simulink model "controlSystem_PowerScope"  (R2021a)
settings: Solver=VariableStepAuto  StartTime=0.0  StopTime=50  RelTol=1e-7
undefined symbols (not defined in the file): initialFuel, maxEngineTemp, maxEngineTorque, maxMotorTemp, maxMotorTorque, maxRegenTorque, motorVoltage, sigbuilder_block
libraries: autolibshared x6, autolibsharedcoupling x3, autolibhevctrlrcommon x2, autolibutils x2, autolibmappedmotor x2, autolibshareddiff x1, autolibtransamt x1, autolibdcdc x1, autolibdatasheetbattery x1, autolibsharedmappedengines x1
(part 3 of 5)

== system controlSystem_PowerScope/Signal Builder ==
  Demux : Demux  Tag=STV Demux  Outputs=3
      settings: DisplayOption=none
  FromWs : FromWorkspace  Tag=STV FromWs  VariableName=tuvar
      SigBuilderData=|
      | common.afterFinalStr = 'Extrapolate'
      | common.sampleTime = 0
      | dataSet.timeRange = [0 50]
      | dataSet.name = 'Group 1'
      | sbobj.Groups.Name = 'Group 1'
      | sbobj.Groups.Signals(1).Name = 'Signal 1'
      | sbobj.Groups.Signals(1).XData = [0 5 5 50]
      | sbobj.Groups.Signals(1).YData = [0 0 1 1]
      | sbobj.Groups.Signals(2).Name = 'Signal 2'
      | sbobj.Groups.Signals(2).XData = [0 50]
      | sbobj.Groups.Signals(2).YData = [0 0]
      | sbobj.Groups.Signals(3).Name = 'Signal 3'
      | sbobj.Groups.Signals(3).XData = [0 5 10 20 25 50]
      | sbobj.Groups.Signals(3).YData = [0 0 1 1 0 0]
      | sbobj.Groups.TimeRange = [0 50]
  Signal 1 : Outport  Tag=STV Outport
  Signal 2 : Outport  Tag=STV Outport  Port=2
  Signal 3 : Outport  Tag=STV Outport  Port=3
  wires:
  Demux/1 -> Signal 1/1
  FromWs/1 -> Demux/1
  Demux/2 -> Signal 2/1
  Demux/3 -> Signal 3/1

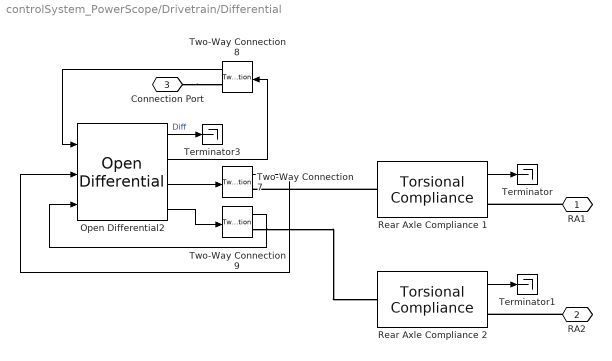
== system controlSystem_PowerScope/Drivetrain/Differential ==
  Open Differential2 : autolibshareddiff/Open Differential  DiffEffModelPopup=Constant  InterpMethod=Linear point-slope  extTamb=off  shaftSwitchMask=To the left of center-line  Ndiff=1  Jd=.025  bd=1e-3  Jw1=.01  bw1=1e-3  Jw2=.01  bw2=1e-3  omegaw1o=0  omegaw2o=0  eta=1  eta_tbl=reshape([0.64 0.76 0.8 0.81 0.83 0.84 0.84 0.56 0.73 0.78 0.8 0.83 0.84 0.84 0.54 0.71 0.77 0.8 0.82 0.84 0.84 0.53 0.71 0.77 0.8 0.83 0.84 0.84 0.51 0.71 0.77 0.8 0.83 0.84 0.85 0.52 0.7 0.77 0.8 0.83 0.84 0.85 0.51 0.71 0.76 0.79 0.83 0.84 0.85 0.5 0.69 0.76 0.79 0.82 0.84 0.85 0.45 0.68 0.75 0.78 0.82 0.84 0.85 0.43 0.67 0.74 0.78 0.81 0.83 0.84 0.38 0.63 0.71 0.75 0.8 0.82 0.83 0.81 0.86 0.88 0.89 0.89 0.89 0.9 0.77 0.85 0.87 0.88 0.89 0.9 0.9 0.72 0.82 0.86 0.87 0.88 0.89 0.9 0.68 0.8 0.84 0.86 0.88 0.89 0.89 0.67 0.8 0.84 0.86 0.88 0.89 0.9 0.67 0.8 0.84 0.86 0.88 0.89 0.9 0.65 0.8 0.84 0.86 0.88 0.89 0.9 0.64 0.79 0.83 0.86 0.88 0.89 0.9 0.63 0.78 0.83 0.86 0.88 0.89 0.9 0.59 0.76 0.82 0.85 0.87 0.89 0.9 0.53 0.73 0.8 0.83 0.86 0.88 0.89], 7, 11, 2)  Trq_bpts=[25, 50, 75, 100, 150, 200, 250]  omega_bpts=[52.4 78.5 105 131 157 183 209 262 314 419 524]  Temp_bpts=[290 358]  Tamb=297.15  maxAbsSpd=5e3  aMode=1
      settings: SourceProductBaseCode=PW,DR,MT,UV,VE
  Rear Axle Compliance 1 : autolibsharedcoupling/Torsional Compliance  port_config=Two-way connection  extInfo=on  k=1e4  b=1e2  theta_o=0  domega_o=0  omega_c=3000  blkID=0  aMode=1
      settings: SourceProductBaseCode=PW,DR,MT,UV,VE
  Rear Axle Compliance 2 : autolibsharedcoupling/Torsional Compliance  port_config=Two-way connection  extInfo=on  k=1e4  b=1e2  theta_o=0  domega_o=0  omega_c=3000  blkID=0  aMode=1
      settings: SourceProductBaseCode=PW,DR,MT,UV,VE
  Terminator : Terminator
  Terminator1 : Terminator
  Terminator3 : Terminator
  Two-Way Connection7 : TwoWayConnection
  Two-Way Connection8 : TwoWayConnection
  Two-Way Connection9 : TwoWayConnection
  RA1 : PMIOPort  Side=Right
  RA2 : PMIOPort  Port=2  Side=Right
  Connection Port : PMIOPort  Port=3  Side=Left
  wires:
  Open Differential2/4 -> Two-Way Connection9/1
  Open Differential2/1 -> Terminator3/1  "Diff"
  Open Differential2/2 -> Two-Way Connection8/1
  Two-Way Connection7/1 -> Open Differential2/2
  Two-Way Connection9/1 -> Open Differential2/3
  Two-Way Connection8/1 -> Open Differential2/1
  Open Differential2/3 -> Two-Way Connection7/1
  Rear Axle Compliance 1/1 -> Terminator/1
  Rear Axle Compliance 2/1 -> Terminator1/1
  connections:
  Two-Way Connection9/RConn1 -- Rear Axle Compliance 2/LConn1
  RA1/RConn1 -- Rear Axle Compliance 1/RConn1
  RA2/RConn1 -- Rear Axle Compliance 2/RConn1
  Rear Axle Compliance 1/LConn1 -- Two-Way Connection7/RConn1
  Connection Port/RConn1 -- Two-Way Connection8/RConn1

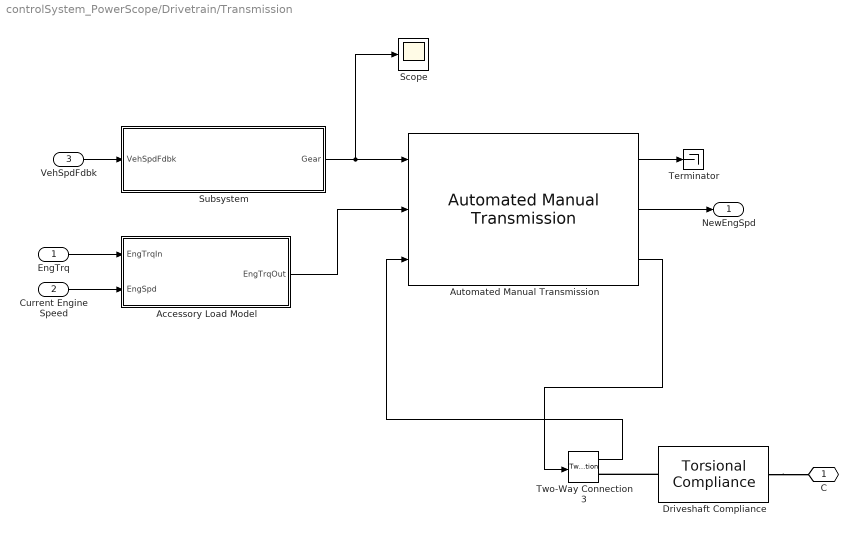
== system controlSystem_PowerScope/Drivetrain/Transmission ==
  EngTrq : Inport
  Current Engine Speed : Inport  Port=2
  VehSpdFdbk : Inport  Port=3
  Accessory Load Model : Subsystem
  Automated Manual Transmission : autolibtransamt/Automated Manual Transmission  VariantControl=0  cntrlType=Ideal integrated controller  TransEffModelPopup=Gear only  Jin=.01  bin=.001  omegain_o=0  G=[0, 1, 2, 3, 4, 5]  Trq_bpts=[25, 50, 75, 100, 150, 200, 250]  omega_bpts=[52.4 78.5 105 131 157 183 209 262 314 419 524]  Temp_bpts=[313 358]  N=[0, 0.4063, 0.5, 0.6071, 0.7308, 0.84]  Jout=[0.01 0.128 0.1 0.062 0.028 0.01]  bout=[.001 .003 .0025 .002 .001 .001]  eta=[0.9, 0.9, 0.9, 0.9, 0.95, 0.95]  eta_tbl=reshape([0.53 0.71 0.77 0.79 0.82 0.82 0.82 0.5 0.7 0.77 0.79 0.82 0.82 0.82 0.54 0.72 0.78 0.81 0.83 0.82 0.82 0.56 0.73 0.79 0.81 0.84 0.82 0.82 0.58 0.74 0.79 0.82 0.84 0.82 0.82 0.57 0.74 0.79 0.82 0.84 0.82 0.82 0.58 0.74 0.79 0.82 0.84 0.82 0.82 0.58 0.74 0.79 0.82 0.84 0.82 0.82 0.57 0.74 0.8 0.82 0.85 0.82 0.82 0.55 0.73 0.78 0.81 0.84 0.82 0.82 0.51 0.71 0.77 0.81 0.84 0.82 0.82 0.53 0.71 0.77 0.79 0.82 0.82 0.82 0.5 0.7 0.77 0.79 0.82 0.82 0.82 0.54 0.72 0.78 0.81 0.83 0.82 0.82 0.56 0.73 0.79 0.81 0.84 0.82 0.82 0.58 0.74 0.79 0.82 0.84 0.82 0.82 0.57 0.74 0.79 0.82 0.84 0.82 0.82 0.58 0.74 0.79 0.82 0.84 0.82 0.82 0.58 0.74 0.79 0.82 0.84 0.82 0.82 0.57 0.74 0.8 0.82 0.85 0.82 0.82 0.55 0.73 0.78 0.81 0.84 0.82 0.82 0.51 0.71 0.77 0.81 0.84 0.82 0.82 0.53 0.71 0.77 0.79 0.82 0.82 0.82 0.5 0.7 0.77 0.79 0.82 0.82 0.82 0.54 0.72 0.78 0.81 0.83 0.82 0.82 0.56 0.73 0.79 0.81 0.84 0.82 0.82 0.58 0.74 0.79 0.82 0.84 0.82 0.82 0.57 0.74 0.79 0.82 0.84 0.82 0.82 0.58 0.74 0.79 0.82 0.84 0.82 0.82 0.58 0.74 0.79 0.82 0.84 0.82 0.82 0.57 0.74 0.8 0.82 0.85 0.82 0.82 0.55 0.73 0.78 0.81 0.84 0.82 0.82 0.51 0.71 0.77 0.81 0.84 0.82 0.82 0.7 0.79 0.82 0.83 0.84 0.84 0.84 0.63 0.76 0.8 0.82 0.83 0.84 0.84 0.58 0.74 0.79 0.81 0.83 0.84 0.84 0.58 0.74 0.79 0.81 0.83 0.84 0.84 0.58 0.74 0.79 0.81 0.84 0.84 0.84 0.57 0.73 0.78 0.81 0.84 0.85 0.84 0.57 0.73 0.79 0.81 0.84 0.85 0.84 0.56 0.73 0.78 0.81 0.83 0.85 0.84 0.55 0.73 0.78 0.81 0.84 0.85 0.84 0.52 0.71 0.77 0.8 0.83 0.85 0.84 0.48 0.69 0.76 0.79 0.83 0.84 0.84 0.64 0.76 0.8 0.81 0.83 0.84 0.84 0.56 0.73 0.78 0.8 0.83 0.84 0.84 0.54 0.71 0.77 0.8 0.82 0.84 0.84 0.53 0.71 0.77 0.8 0.83 0.84 0.84 0.51 0.71 0.77 0.8 0.83 0.84 0.85 0.52 0.7 0.77 0.8 0.83 0.84 0.85 0.51 0.71 0.76 0.79 0.83 0.84 0.85 0.5 0.69 0.76 0.79 0.82 0.84 0.85 0.45 0.68 0.75 0.78 0.82 0.84 0.85 0.43 0.67 0.74 0.78 0.81 0.83 0.84 0.38 0.63 0.71 0.75 0.8 0.82 0.83 0.65 0.79 0.84 0.85 0.88 0.89 0.89 0.56 0.75 0.81 0.83 0.86 0.88 0.89 0.52 0.72 0.79 0.83 0.86 0.88 0.88 0.51 0.72 0.79 0.83 0.86 0.88 0.89 0.49 0.71 0.78 0.82 0.86 0.88 0.89 0.47 0.7 0.78 0.82 0.86 0.87 0.88 0.45 0.69 0.77 0.81 0.85 0.87 0.88 0.4 0.67 0.75 0.8 0.84 0.86 0.88 0.3 0.64 0.73 0.78 0.83 0.86 0.87 0.17 0.55 0.67 0.73 0.8 0.83 0.85 0.089 0.45 0.61 0.69 0.77 0.81 0.83 0.61 0.75 0.82 0.84 0.87 0.87 0.88 0.54 0.73 0.8 0.82 0.86 0.87 0.88 0.51 0.71 0.79 0.82 0.86 0.87 0.88 0.52 0.72 0.79 0.82 0.86 0.87 0.89 0.52 0.72 0.8 0.83 0.86 0.88 0.89 0.53 0.72 0.79 0.82 0.86 0.87 0.89 0.5 0.7 0.78 0.82 0.86 0.88 0.88 0.46 0.69 0.77 0.81 0.85 0.87 0.88 0.4 0.67 0.75 0.8 0.83 0.86 0.88 0.33 0.64 0.73 0.78 0.83 0.85 0.87 0.33 0.64 0.73 0.78 0.83 0.85 0.87 0.78 0.85 0.87 0.88 0.89 0.89 0.89 0.73 0.83 0.86 0.88 0.89 0.89 0.89 0.72 0.83 0.86 0.88 0.89 0.89 0.89 0.72 0.83 0.87 0.89 0.9 0.89 0.89 0.72 0.83 0.87 0.88 0.9 0.89 0.89 0.71 0.83 0.87 0.88 0.9 0.89 0.89 0.71 0.83 0.86 0.88 0.9 0.89 0.89 0.7 0.82 0.86 0.88 0.9 0.89 0.89 0.69 0.82 0.86 0.88 0.9 0.89 0.89 0.67 0.81 0.86 0.88 0.9 0.89 0.89 0.63 0.79 0.85 0.87 0.89 0.89 0.89 0.78 0.85 0.87 0.88 0.89 0.89 0.89 0.73 0.83 0.86 0.88 0.89 0.89 0.89 0.72 0.83 0.86 0.88 0.89 0.89 0.89 0.72 0.83 0.87 0.89 0.9 0.89 0.89 0.72 0.83 0.87 0.88 0.9 0.89 0.89 0.71 0.83 0.87 0.88 0.9 0.89 0.89 0.71 0.83 0.86 0.88 0.9 0.89 0.89 0.7 0.82 0.86 0.88 0.9 0.89 0.89 0.69 0.82 0.86 0.88 0.9 0.89 0.89 0.67 0.81 0.86 0.88 0.9 0.89 0.89 0.63 0.79 0.85 0.87 0.89 0.89 0.89 0.78 0.85 0.87 0.88 0.89 0.89 0.89 0.73 0.83 0.86 0.88 0.89 0.89 0.89 0.72 0.83 0.86 0.88 0.89 0.89 0.89 0.72 0.83 0.87 0.89 0.9 0.89 0.89 0.72 0.83 0.87 0.88 0.9 0.89 0.89 0.71 0.83 0.87 0.88 0.9 0.89 0.89 0.71 0.83 0.86 0.88 0.9 0.89 0.89 0.7 0.82 0.86 0.88 0.9 0.89 0.89 0.69 0.82 0.86 0.88 0.9 0.89 0.89 0.67 0.81 0.86 0.88 0.9 0.89 0.89 0.63 0.79 0.85 0.87 0.89 0.89 0.89 0.82 0.87 0.88 0.89 0.89 0.89 0.89 0.81 0.87 0.89 0.89 0.9 0.9 0.89 0.76 0.85 0.87 0.89 0.9 0.89 0.89 0.72 0.83 0.86 0.88 0.89 0.89 0.89 0.72 0.83 0.86 0.88 0.89 0.9 0.89 0.71 0.82 0.86 0.88 0.89 0.9 ...(+1314 chars))  omegaout_o=0  G_o=0  tauc=.02  ts=.25  tc=.5  R=.2  K_c=5e3  mus=0.6  muk=0.4  ClutchLocked=off  SynchLocked=off  maxAbsSpd=5e3
      settings: SourceProductBaseCode=PW
  Driveshaft Compliance : autolibsharedcoupling/Torsional Compliance  port_config=Two-way connection  extInfo=off  k=1e4  b=1e2  theta_o=0  domega_o=0  omega_c=3000  blkID=0  aMode=1
      settings: SourceProductBaseCode=PW,DR,MT,UV,VE
  Scope : Scope
  Subsystem : Subsystem
  Terminator : Terminator
  Two-Way Connection3 : TwoWayConnection
  C : PMIOPort  Side=Right
  NewEngSpd : Outport
  wires:
  Automated Manual Transmission/2 -> NewEngSpd/1
  Accessory Load Model/1(EngTrqOut) -> Automated Manual Transmission/2
  Current Engine Speed/1 -> Accessory Load Model/2(EngSpd)
  Two-Way Connection3/1 -> Automated Manual Transmission/3
  EngTrq/1 -> Accessory Load Model/1(EngTrqIn)
  Automated Manual Transmission/3 -> Two-Way Connection3/1
  Subsystem/1(Gear) -> Scope/1, Automated Manual Transmission/1
  VehSpdFdbk/1 -> Subsystem/1(VehSpdFdbk)
  Automated Manual Transmission/1 -> Terminator/1
  connections:
  Driveshaft Compliance/RConn1 -- C/RConn1
  Driveshaft Compliance/LConn1 -- Two-Way Connection3/RConn1

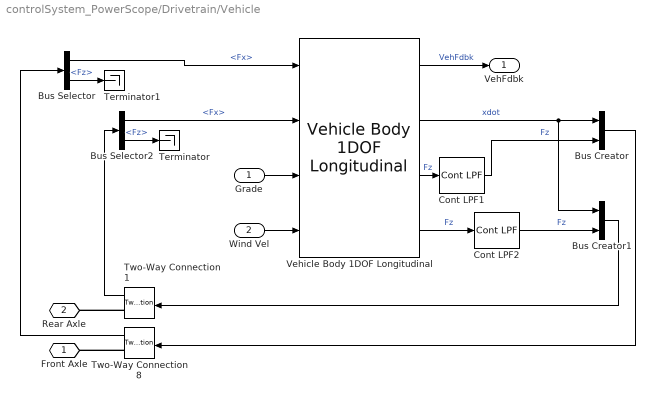
== system controlSystem_PowerScope/Drivetrain/Vehicle ==
  Grade : Inport  Unit=deg
  Wind Vel : Inport  Port=2  Unit=m/s
  Bus Creator : BusCreator  Inputs=2
  Bus Creator1 : BusCreator  Inputs=2
  Bus Selector : BusSelector  OutputSignals=Fx,Fz
  Bus Selector2 : BusSelector  OutputSignals=Fx,Fz
  Cont LPF1 : autolibutils/Cont LPF  wc=10  aMode=aMode
      settings: SourceProductBaseCode=PW,DR,MT,UV,VE
  Cont LPF2 : autolibutils/Cont LPF  wc=10  aMode=aMode
      settings: SourceProductBaseCode=PW,DR,MT,UV,VE
  Terminator : Terminator
  Terminator1 : Terminator
  Two-Way Connection1 : TwoWayConnection
  Two-Way Connection8 : TwoWayConnection
  Vehicle Body 1DOF Longitudinal : autolibshared/Vehicle Body 1DOF Longitudinal  VariantControl=SL  extFMode=off  extMMode=off  extTamb=off  wind3D=off  aMode=1  NF=2  NR=2  m=300  a=0.7  b=0.5  h=0.15  Cd=.3  Cl=0  Cpm=0  Af=1  x_o=0  xdot_o=0  Pabs=101325  T=290  g=9.81
      settings: SourceProductBaseCode=PW,DR,MT,UV,VE
  Front Axle : PMIOPort  Side=Left
  Rear Axle : PMIOPort  Port=2  Side=Left
  VehFdbk : Outport
  wires:
  Vehicle Body 1DOF Longitudinal/3 -> Cont LPF1/1  "Fz"
  Vehicle Body 1DOF Longitudinal/2 -> Bus Creator1/1, Bus Creator/1  "xdot"
  Two-Way Connection8/1 -> Bus Selector/1
  Vehicle Body 1DOF Longitudinal/4 -> Cont LPF2/1  "Fz"
  Grade/1 -> Vehicle Body 1DOF Longitudinal/3
  Wind Vel/1 -> Vehicle Body 1DOF Longitudinal/4
  Bus Creator/1 -> Two-Way Connection8/1
  Bus Creator1/1 -> Two-Way Connection1/1
  Bus Selector/1 -> Vehicle Body 1DOF Longitudinal/1  "<Fx>"
  Bus Selector2/1 -> Vehicle Body 1DOF Longitudinal/2  "<Fx>"
  Two-Way Connection1/1 -> Bus Selector2/1
  Vehicle Body 1DOF Longitudinal/1 -> VehFdbk/1  "VehFdbk"
  Bus Selector2/2 -> Terminator/1  "<Fz>"
  Bus Selector/2 -> Terminator1/1  "<Fz>"
  Cont LPF1/1 -> Bus Creator/2  "Fz"
  Cont LPF2/1 -> Bus Creator1/2  "Fz"
  connections:
  Two-Way Connection8/RConn1 -- Front Axle/RConn1
  Two-Way Connection1/RConn1 -- Rear Axle/RConn1
